simulink model "IEEE14_case"  (R2024b)
settings: Solver=FixedStepAuto  StartTime=0  StopTime=2  FixedStep=1e-7  RelTol=1e-3
values from neighbouring files (symbols this model uses):
  GFL_15_Bva = 0.009    [IEEE14_parameters.m]
  GFL_15_C_bus_pu = 7.179419    [IEEE14_parameters.m]
  GFL_15_f0 = 60    [IEEE14_parameters.m]
  GFL_15_I_id = 691.26967    [IEEE14_parameters.m]
  GFL_15_I_iq = 691.26967    [IEEE14_parameters.m]
  GFL_15_I_od = 45.2207    [IEEE14_parameters.m]
  GFL_15_I_oq = 45.2207    [IEEE14_parameters.m]
  GFL_15_I_pll = 0.78    [IEEE14_parameters.m]
  GFL_15_Kdi = 0.09    [IEEE14_parameters.m]
  GFL_15_Kdo = 0.9    [IEEE14_parameters.m]
  GFL_15_Kqi = 0.09    [IEEE14_parameters.m]
  GFL_15_Kqo = 0.9    [IEEE14_parameters.m]
  GFL_15_Lg_pu = 0.631447    [IEEE14_parameters.m]
  GFL_15_mode = 1    [IEEE14_parameters.m]
  GFL_15_P_id = 3.7166    [IEEE14_parameters.m]
  GFL_15_P_iq = 3.7166    [IEEE14_parameters.m]
  GFL_15_P_od = 0.4798    [IEEE14_parameters.m]
  GFL_15_P_oq = 0.4798    [IEEE14_parameters.m]
  GFL_15_P_pll = 290.42    [IEEE14_parameters.m]
  GFL_15_Qe_ref = 0.2    [IEEE14_parameters.m]
  GFL_15_Rg_pu = 0.024016    [IEEE14_parameters.m]
  GFL_15_Sbase = 1.000000e+4    (= 10000)    [IEEE14_parameters.m]
  GFL_15_Tdi = 0.01    [IEEE14_parameters.m]
  GFL_15_Tdo = 0.2    [IEEE14_parameters.m]
  GFL_15_Tqi = 0.01    [IEEE14_parameters.m]
  GFL_15_Tqo = 0.2    [IEEE14_parameters.m]
  GFL_15_Vbase = 380    [IEEE14_parameters.m]
  GFL_15_Vdc_ref = 1.011475    [IEEE14_parameters.m]
  GFL_15_Vdcbase = 700    [IEEE14_parameters.m]
  GFL_15_vq_ref = 0    [IEEE14_parameters.m]
  GFL_16_Bva = 0.002    [IEEE14_parameters.m]
  GFL_16_C_bus_pu = 7.179419    [IEEE14_parameters.m]
  GFL_16_f0 = 60    [IEEE14_parameters.m]
  GFL_16_I_id = 691.26967    [IEEE14_parameters.m]
  GFL_16_I_iq = 691.26967    [IEEE14_parameters.m]
  GFL_16_I_od = 45.2207    [IEEE14_parameters.m]
  GFL_16_I_oq = 45.2207    [IEEE14_parameters.m]
  GFL_16_I_pll = 0.78    [IEEE14_parameters.m]
  GFL_16_Kdi = 0.05    [IEEE14_parameters.m]
  GFL_16_Kdo = 0.5    [IEEE14_parameters.m]
  GFL_16_Kqi = 0.05    [IEEE14_parameters.m]
  GFL_16_Kqo = 0.5    [IEEE14_parameters.m]
  GFL_16_Lg_pu = 0.631447    [IEEE14_parameters.m]
  GFL_16_mode = 1    [IEEE14_parameters.m]
  GFL_16_P_id = 3.7166    [IEEE14_parameters.m]
  GFL_16_P_iq = 3.7166    [IEEE14_parameters.m]
  GFL_16_P_od = 0.4798    [IEEE14_parameters.m]
  GFL_16_P_oq = 0.4798    [IEEE14_parameters.m]
  GFL_16_P_pll = 290.42    [IEEE14_parameters.m]
  GFL_16_Qe_ref = 0.2    [IEEE14_parameters.m]
  GFL_16_Rg_pu = 0.024016    [IEEE14_parameters.m]
  GFL_16_Sbase = 1.000000e+4    (= 10000)    [IEEE14_parameters.m]
  GFL_16_Tdi = 0.01    [IEEE14_parameters.m]
  GFL_16_Tdo = 0.2    [IEEE14_parameters.m]
  GFL_16_Tqi = 0.01    [IEEE14_parameters.m]
  GFL_16_Tqo = 0.2    [IEEE14_parameters.m]
  GFL_16_Vbase = 380    [IEEE14_parameters.m]
  GFL_16_Vdc_ref = 1.01144    [IEEE14_parameters.m]
  GFL_16_Vdcbase = 700    [IEEE14_parameters.m]
  GFL_16_vq_ref = 0    [IEEE14_parameters.m]
  GFL_17_Bva = 0.002    [IEEE14_parameters.m]
  GFL_17_C_bus_pu = 7.179419    [IEEE14_parameters.m]
  GFL_17_f0 = 60    [IEEE14_parameters.m]
  GFL_17_I_id = 691.26967    [IEEE14_parameters.m]
  GFL_17_I_iq = 691.26967    [IEEE14_parameters.m]
  GFL_17_I_od = 45.2207    [IEEE14_parameters.m]
  GFL_17_I_oq = 45.2207    [IEEE14_parameters.m]
  GFL_17_I_pll = 0.78    [IEEE14_parameters.m]
  GFL_17_Kdi = 0.05    [IEEE14_parameters.m]
  GFL_17_Kdo = 0.5    [IEEE14_parameters.m]
  GFL_17_Kqi = 0.05    [IEEE14_parameters.m]
  GFL_17_Kqo = 0.5    [IEEE14_parameters.m]
  GFL_17_Lg_pu = 0.631447    [IEEE14_parameters.m]
  GFL_17_mode = 1    [IEEE14_parameters.m]
  GFL_17_P_id = 3.7166    [IEEE14_parameters.m]
  GFL_17_P_iq = 3.7166    [IEEE14_parameters.m]
  GFL_17_P_od = 0.4798    [IEEE14_parameters.m]
  GFL_17_P_oq = 0.4798    [IEEE14_parameters.m]
  GFL_17_P_pll = 290.42    [IEEE14_parameters.m]
  GFL_17_Qe_ref = 0.2    [IEEE14_parameters.m]
  GFL_17_Rg_pu = 0.024016    [IEEE14_parameters.m]
  GFL_17_Sbase = 1.000000e+4    (= 10000)    [IEEE14_parameters.m]
  GFL_17_Tdi = 0.01    [IEEE14_parameters.m]
  GFL_17_Tdo = 0.2    [IEEE14_parameters.m]
  GFL_17_Tqi = 0.01    [IEEE14_parameters.m]
  GFL_17_Tqo = 0.2    [IEEE14_parameters.m]
  GFL_17_Vbase = 380    [IEEE14_parameters.m]
  GFL_17_Vdc_ref = 1.011632    [IEEE14_parameters.m]
  GFL_17_Vdcbase = 700    [IEEE14_parameters.m]
  GFL_17_vq_ref = 0    [IEEE14_parameters.m]
  GFL_18_Bva = 0.002    [IEEE14_parameters.m]
  GFL_18_C_bus_pu = 7.179419    [IEEE14_parameters.m]
  GFL_18_f0 = 60    [IEEE14_parameters.m]
  GFL_18_I_id = 691.26967    [IEEE14_parameters.m]
  GFL_18_I_iq = 691.26967    [IEEE14_parameters.m]
  GFL_18_I_od = 45.2207    [IEEE14_parameters.m]
  GFL_18_I_oq = 45.2207    [IEEE14_parameters.m]
  GFL_18_I_pll = 0.78    [IEEE14_parameters.m]
  GFL_18_Kdi = 0.05    [IEEE14_parameters.m]
  GFL_18_Kdo = 0.5    [IEEE14_parameters.m]
  GFL_18_Kqi = 0.05    [IEEE14_parameters.m]
  GFL_18_Kqo = 0.5    [IEEE14_parameters.m]
  GFL_18_Lg_pu = 0.631447    [IEEE14_parameters.m]
  GFL_18_mode = 1    [IEEE14_parameters.m]
  GFL_18_P_id = 3.7166    [IEEE14_parameters.m]
  GFL_18_P_iq = 3.7166    [IEEE14_parameters.m]
  GFL_18_P_od = 0.4798    [IEEE14_parameters.m]
  GFL_18_P_oq = 0.4798    [IEEE14_parameters.m]
  GFL_18_P_pll = 290.42    [IEEE14_parameters.m]
  GFL_18_Qe_ref = 0.2    [IEEE14_parameters.m]
  GFL_18_Rg_pu = 0.024016    [IEEE14_parameters.m]
  GFL_18_Sbase = 1.000000e+4    (= 10000)    [IEEE14_parameters.m]
  GFL_18_Tdi = 0.01    [IEEE14_parameters.m]
  GFL_18_Tdo = 0.2    [IEEE14_parameters.m]
  GFL_18_Tqi = 0.01    [IEEE14_parameters.m]
  GFL_18_Tqo = 0.2    [IEEE14_parameters.m]
  GFL_18_Vbase = 380    [IEEE14_parameters.m]
  GFL_18_Vdc_ref = 1.011572    [IEEE14_parameters.m]
  GFL_18_Vdcbase = 700    [IEEE14_parameters.m]
  GFL_18_vq_ref = 0    [IEEE14_parameters.m]
  ... (+180 more)
(part 16 of 25)

== system IEEE14_case/SG_D_1/d_psi_d_SG_D_1_block ==
  note: d_psi_d_SG_D_1 in case14gfl
      | $2\,\pi \,f_{0}\,\left(v_{d,\mathrm{SG},D,1}\,\sin\left(\theta _{\mathrm{SG},D,1}\right)-v_{q,\mathrm{SG},D,1}\,\cos\left(\theta _{\mathrm{SG},D,1}\right)+\frac{R_{a}\,\left(\frac{\psi _{\mathrm{1d},\mathrm{SG},D,1}\,\left(x_{\mathrm{dd}}-x_{\mathrm{ddd}}\right)}{x_{\mathrm{dd}}-x_{l}}-\psi _{d,\mathrm{SG},D,1}+\frac{\psi _{\mathrm{fd},\mathrm{SG},D,1}\,\left(x_{\mathrm{ddd}}-x_{l}\right)}{x_{\mathrm{dd}}-x_{l}}\right)}{x_{\mathrm{ddd}}}+\frac{\psi _{q,\mathrm{SG},D,1}\,w_{\mathrm{SG},D,1}}{2\,f_{0}\,\pi }\right)$
      | Automatically generated on 2025-10-09 21:29:31 .
  State_psi_1d_SG_D_1_69d00 : Inport
  State_psi_d_SG_D_1_b0cbd : Inport  Port=2
  State_psi_fd_SG_D_1_aad83 : Inport  Port=3
  Input_v_d_SG_D_1_751e0 : Inport  Port=4
  State_theta_SG_D_1_5b2d6 : Inport  Port=5
  Input_v_q_SG_D_1_569c6 : Inport  Port=6
  State_theta_SG_D_1_7d7a3 : Inport  Port=7
  State_psi_q_SG_D_1_339cd : Inport  Port=8
  State_w_SG_D_1_7866a : Inport  Port=9
  Add_56184 : Sum
  Add_be544 : Sum
  Constant_-1_51278 : Constant  Value=-1
  Constant_-2.0_38dac : Constant  Value=-2.0
  Constant_2.0_c29de : Constant  Value=2.0
  Constant_R_a_cf787 : Constant  Value=R_a
  Constant_f0_76831 : Constant  Value=f0
  Constant_f0_cb811 : Constant  Value=f0
  Constant_pi_8af64 : Constant  Value=pi
  Constant_pi_fa2ea : Constant  Value=pi
  Constant_x_dd_7e7b6 : Constant  Value=x_dd
  Constant_x_dd_812da : Constant  Value=x_dd
  Constant_x_dd_b764a : Constant  Value=x_dd
  Constant_x_ddd_361c2 : Constant  Value=x_ddd
  Constant_x_ddd_731d1 : Constant  Value=x_ddd
  Constant_x_ddd_f45d6 : Constant  Value=x_ddd
  Constant_x_l_01895 : Constant  Value=x_l
  Constant_x_l_16bb1 : Constant  Value=x_l
  Constant_x_l_4d5b7 : Constant  Value=x_l
  Divide_0c8f7 : Product  Inputs=*/
  Divide_7e30b : Product  Inputs=*/
  Divide_b7777 : Product  Inputs=*/
  Divide_c3a43 : Product  Inputs=*/
  MathFunc_cos_3b064 : Trigonometry  Operator=cos
  MathFunc_sin_7ab60 : Trigonometry
  Product_22a26 : Product
  Product_40b9a : Product
  Product_4496c : Product
  Product_63206 : Product
  Product_9a24b : Product
  Product_ac20e : Product
  Product_b01b2 : Product
  Product_b1bbd : Product
  Product_b9918 : Product
  Product_d2dbc : Product
  Product_d68ab : Product
  Product_e52bf : Product
  Subtract_0ab8d : Sum  Inputs=+-
  Subtract_2360f : Sum  Inputs=+-
  Subtract_60414 : Sum  Inputs=+-
  Subtract_87491 : Sum  Inputs=+-
  Subtract_a23d2 : Sum  Inputs=+-
  Subtract_c2635 : Sum  Inputs=+-
  Subtract_ccf2d : Sum  Inputs=+-
  Blockout_d_psi_d_SG_D_1_2cdbf : Outport
  wires:
  Add_be544/1 -> Subtract_87491/1
  Product_9a24b/1 -> Divide_c3a43/1
  Subtract_ccf2d/1 -> Product_9a24b/2
  Divide_c3a43/1 -> Add_be544/1
  Product_e52bf/1 -> Product_9a24b/1
  Constant_x_ddd_361c2/1 -> Subtract_ccf2d/2
  Constant_x_dd_812da/1 -> Subtract_ccf2d/1
  State_psi_1d_SG_D_1_69d00/1 -> Product_e52bf/2
  Constant_-1_51278/1 -> Product_e52bf/1
  Product_ac20e/1 -> Divide_b7777/1
  Constant_x_l_4d5b7/1 -> Subtract_c2635/2
  State_psi_d_SG_D_1_b0cbd/1 -> Add_be544/2
  Constant_x_dd_b764a/1 -> Subtract_c2635/1
  Constant_x_ddd_731d1/1 -> Subtract_a23d2/1
  Constant_x_l_01895/1 -> Subtract_a23d2/2
  Subtract_c2635/1 -> Divide_c3a43/2
  State_psi_fd_SG_D_1_aad83/1 -> Product_ac20e/1
  Constant_x_ddd_f45d6/1 -> Divide_0c8f7/2
  Subtract_a23d2/1 -> Product_ac20e/2
  Product_d68ab/1 -> Subtract_0ab8d/2
  Constant_x_dd_7e7b6/1 -> Subtract_2360f/1
  Constant_x_l_16bb1/1 -> Subtract_2360f/2
  Subtract_2360f/1 -> Divide_b7777/2
  Divide_b7777/1 -> Subtract_87491/2
  Constant_R_a_cf787/1 -> Product_63206/1
  Subtract_87491/1 -> Product_63206/2
  MathFunc_cos_3b064/1 -> Product_4496c/2
  State_theta_SG_D_1_5b2d6/1 -> MathFunc_sin_7ab60/1
  Divide_0c8f7/1 -> Subtract_0ab8d/1
  Product_63206/1 -> Divide_0c8f7/1
  MathFunc_sin_7ab60/1 -> Product_d68ab/2
  Input_v_d_SG_D_1_751e0/1 -> Product_d68ab/1
  Product_b9918/1 -> Blockout_d_psi_d_SG_D_1_2cdbf/1
  Product_d2dbc/1 -> Product_b9918/1
  Product_22a26/1 -> Product_d2dbc/1
  State_theta_SG_D_1_7d7a3/1 -> MathFunc_cos_3b064/1
  Constant_2.0_c29de/1 -> Product_40b9a/1
  Constant_pi_fa2ea/1 -> Product_40b9a/2
  Input_v_q_SG_D_1_569c6/1 -> Product_4496c/1
  Constant_f0_76831/1 -> Product_d2dbc/2
  State_psi_q_SG_D_1_339cd/1 -> Product_b1bbd/1
  State_w_SG_D_1_7866a/1 -> Product_b1bbd/2
  Product_40b9a/1 -> Product_b01b2/1
  Constant_pi_8af64/1 -> Product_22a26/2
  Constant_f0_cb811/1 -> Product_b01b2/2
  Constant_-2.0_38dac/1 -> Product_22a26/1
  Add_56184/1 -> Subtract_60414/1
  Subtract_0ab8d/1 -> Add_56184/1
  Product_4496c/1 -> Add_56184/2
  Product_b1bbd/1 -> Divide_7e30b/1
  Product_b01b2/1 -> Divide_7e30b/2
  Divide_7e30b/1 -> Subtract_60414/2
  Subtract_60414/1 -> Product_b9918/2

== system IEEE14_case/SG_D_1/d_psi_fd_SG_D_1_block ==
  note: d_psi_fd_SG_D_1 in case14gfl
      | $-\frac{\psi _{\mathrm{fd},\mathrm{SG},D,1}-E_{\mathrm{fd},\mathrm{SG},D,1}+\left(x_{d}-x_{\mathrm{dd}}\right)\,\left(\frac{\frac{\psi _{\mathrm{1d},\mathrm{SG},D,1}\,\left(x_{\mathrm{dd}}-x_{\mathrm{ddd}}\right)}{x_{\mathrm{dd}}-x_{l}}-\psi _{d,\mathrm{SG},D,1}+\frac{\psi _{\mathrm{fd},\mathrm{SG},D,1}\,\left(x_{\mathrm{ddd}}-x_{l}\right)}{x_{\mathrm{dd}}-x_{l}}}{x_{\mathrm{ddd}}}-\frac{\left(x_{\mathrm{dd}}-x_{\mathrm{ddd}}\right)\,\left(\psi _{\mathrm{1d},\mathrm{SG},D,1}-\psi _{\mathrm{fd},\mathrm{SG},D,1}+\frac{\left(x_{\mathrm{dd}}-x_{l}\right)\,\left(\frac{\psi _{\mathrm{1d},\mathrm{SG},D,1}\,\left(x_{\mathrm{dd}}-x_{\mathrm{ddd}}\right)}{x_{\mathrm{dd}}-x_{l}}-\psi _{d,\mathrm{SG},D,1}+\frac{\psi _{\mathrm{fd},\mathrm{SG},D,1}\,\left(x_{\mathrm{ddd}}-x_{l}\right)}{x_{\mathrm{dd}}-x_{l}}\right)}{x_{\mathrm{ddd}}}\right)}{{\left(x_{\mathrm{dd}}-x_{l}\right)}^2}\right)}{T_{\mathrm{dd}}}$
      | Automatically generated on 2025-10-09 21:29:56 .
  State_E_fd_SG_D_1_05819 : Inport
  State_psi_fd_SG_D_1_8f7d3 : Inport  Port=2
  State_psi_1d_SG_D_1_1898e : Inport  Port=3
  State_psi_fd_SG_D_1_d976b : Inport  Port=4
  State_psi_1d_SG_D_1_f6ad7 : Inport  Port=5
  State_psi_d_SG_D_1_eef22 : Inport  Port=6
  State_psi_fd_SG_D_1_c7a2f : Inport  Port=7
  State_psi_1d_SG_D_1_2c9f9 : Inport  Port=8
  State_psi_d_SG_D_1_5418d : Inport  Port=9
  State_psi_fd_SG_D_1_86724 : Inport  Port=10
  Add_0e10e : Sum
  Add_855f0 : Sum
  Constant_-1_2c57e : Constant  Value=-1
  Constant_-1_a28a2 : Constant  Value=-1
  Constant_-1_c60db : Constant  Value=-1
  Constant_2.0_ead1b : Constant  Value=2.0
  Constant_T_dd_4fac4 : Constant  Value=T_dd
  Constant_x_d_dd175 : Constant  Value=x_d
  Constant_x_dd_048c0 : Constant  Value=x_dd
  Constant_x_dd_0c681 : Constant  Value=x_dd
  Constant_x_dd_17d74 : Constant  Value=x_dd
  Constant_x_dd_1bbdd : Constant  Value=x_dd
  Constant_x_dd_2d3b2 : Constant  Value=x_dd
  Constant_x_dd_32bd9 : Constant  Value=x_dd
  Constant_x_dd_778d2 : Constant  Value=x_dd
  Constant_x_dd_c0a9a : Constant  Value=x_dd
  Constant_x_dd_d296d : Constant  Value=x_dd
  Constant_x_dd_f5264 : Constant  Value=x_dd
  Constant_x_ddd_147e2 : Constant  Value=x_ddd
  Constant_x_ddd_27727 : Constant  Value=x_ddd
  Constant_x_ddd_30073 : Constant  Value=x_ddd
  Constant_x_ddd_77236 : Constant  Value=x_ddd
  Constant_x_ddd_7c972 : Constant  Value=x_ddd
  Constant_x_ddd_8e231 : Constant  Value=x_ddd
  Constant_x_ddd_dc7b0 : Constant  Value=x_ddd
  Constant_x_l_2ab6b : Constant  Value=x_l
  Constant_x_l_30b80 : Constant  Value=x_l
  Constant_x_l_71782 : Constant  Value=x_l
  Constant_x_l_74cf2 : Constant  Value=x_l
  Constant_x_l_98a55 : Constant  Value=x_l
  Constant_x_l_9e494 : Constant  Value=x_l
  Constant_x_l_a6392 : Constant  Value=x_l
  Constant_x_l_beb3a : Constant  Value=x_l
  Divide_01689 : Product  Inputs=*/
  Divide_0f83a : Product  Inputs=*/
  Divide_6a9fb : Product  Inputs=*/
  Divide_7fd4b : Product  Inputs=*/
  Divide_9001b : Product  Inputs=*/
  Divide_a851a : Product  Inputs=*/
  Divide_b92f6 : Product  Inputs=*/
  Divide_fdf02 : Product  Inputs=*/
  Power_7840a : Math  Operator=pow
  Product_16821 : Product
  Product_1a66a : Product
  Product_2f431 : Product
  Product_6b392 : Product
  Product_7d54a : Product
  Product_b5b20 : Product
  Product_b5cc8 : Product
  Product_b7127 : Product
  Product_d3415 : Product
  Product_f7a96 : Product
  Subtract_0cd1e : Sum  Inputs=+-
  Subtract_2a961 : Sum  Inputs=+-
  Subtract_3bb19 : Sum  Inputs=+-
  Subtract_4453c : Sum  Inputs=+-
  Subtract_469f7 : Sum  Inputs=+-
  Subtract_562ce : Sum  Inputs=+-
  Subtract_63680 : Sum  Inputs=+-
  Subtract_65ab3 : Sum  Inputs=+-
  Subtract_6a7c7 : Sum  Inputs=+-
  Subtract_6faa6 : Sum  Inputs=+-
  Subtract_72a4d : Sum  Inputs=+-
  Subtract_73178 : Sum  Inputs=+-
  Subtract_80272 : Sum  Inputs=+-
  Subtract_9f379 : Sum  Inputs=+-
  Subtract_b24c4 : Sum  Inputs=+-
  Subtract_b29f2 : Sum  Inputs=+-
  Subtract_cbbe3 : Sum  Inputs=+-
  Subtract_db76e : Sum  Inputs=+-
  Subtract_ff79e : Sum  Inputs=+-
  Blockout_d_psi_fd_SG_D_1_936e9 : Outport
  wires:
  State_psi_d_SG_D_1_eef22/1 -> Add_855f0/2
  Constant_x_dd_17d74/1 -> Subtract_73178/1
  Product_2f431/1 -> Divide_01689/1
  Subtract_65ab3/1 -> Product_2f431/2
  Subtract_6faa6/1 -> Product_d3415/2
  Product_b5b20/1 -> Product_2f431/1
  Constant_x_dd_f5264/1 -> Subtract_65ab3/1
  Constant_x_l_30b80/1 -> Subtract_3bb19/2
  Constant_-1_2c57e/1 -> Product_b5b20/1
  Subtract_3bb19/1 -> Product_d3415/1
  Constant_x_l_71782/1 -> Subtract_73178/2
  Constant_x_ddd_27727/1 -> Subtract_65ab3/2
  State_psi_1d_SG_D_1_f6ad7/1 -> Product_b5b20/2
  Constant_x_ddd_dc7b0/1 -> Subtract_63680/1
  Constant_x_l_a6392/1 -> Subtract_63680/2
  State_E_fd_SG_D_1_05819/1 -> Subtract_2a961/1
  Divide_01689/1 -> Add_855f0/1
  Subtract_73178/1 -> Divide_01689/2
  State_psi_fd_SG_D_1_c7a2f/1 -> Product_1a66a/1
  Constant_x_ddd_8e231/1 -> Divide_7fd4b/2
  Subtract_63680/1 -> Product_1a66a/2
  Constant_x_dd_1bbdd/1 -> Subtract_4453c/1
  Constant_x_dd_048c0/1 -> Subtract_0cd1e/1
  State_psi_fd_SG_D_1_8f7d3/1 -> Subtract_2a961/2
  Constant_x_l_2ab6b/1 -> Subtract_4453c/2
  Product_1a66a/1 -> Divide_b92f6/1
  Constant_-1_c60db/1 -> Product_b5cc8/1
  Subtract_4453c/1 -> Divide_b92f6/2
  Constant_x_dd_d296d/1 -> Subtract_3bb19/1
  Add_855f0/1 -> Subtract_6faa6/1
  Constant_x_l_9e494/1 -> Subtract_0cd1e/2
  Divide_b92f6/1 -> Subtract_6faa6/2
  Divide_0f83a/1 -> Subtract_9f379/1
  Constant_-1_a28a2/1 -> Product_7d54a/1
  State_psi_1d_SG_D_1_2c9f9/1 -> Product_7d54a/2
  Constant_x_dd_c0a9a/1 -> Subtract_db76e/1
  Subtract_80272/1 -> Product_b5cc8/2
  Constant_x_ddd_30073/1 -> Subtract_db76e/2
  Product_7d54a/1 -> Product_16821/1
  Constant_2.0_ead1b/1 -> Power_7840a/2
  Product_16821/1 -> Divide_9001b/1
  Subtract_9f379/1 -> Product_6b392/2
  Subtract_db76e/1 -> Product_16821/2
  State_psi_d_SG_D_1_5418d/1 -> Add_0e10e/2
  Constant_x_dd_32bd9/1 -> Subtract_6a7c7/1
  Constant_x_l_beb3a/1 -> Subtract_6a7c7/2
  Constant_x_dd_0c681/1 -> Subtract_80272/1
  Divide_7fd4b/1 -> Subtract_562ce/2
  Constant_x_ddd_147e2/1 -> Subtract_b29f2/1
  Constant_x_ddd_7c972/1 -> Subtract_80272/2
  Constant_x_l_98a55/1 -> Subtract_b29f2/2
  Subtract_b29f2/1 -> Product_f7a96/2
  State_psi_1d_SG_D_1_1898e/1 -> Subtract_cbbe3/1
  Product_f7a96/1 -> Divide_6a9fb/1
  State_psi_fd_SG_D_1_d976b/1 -> Subtract_cbbe3/2
  State_psi_fd_SG_D_1_86724/1 -> Product_f7a96/1
  Product_d3415/1 -> Divide_7fd4b/1
  Divide_9001b/1 -> Add_0e10e/1
  Subtract_6a7c7/1 -> Divide_9001b/2
  Constant_x_dd_778d2/1 -> Subtract_72a4d/1
  Constant_x_l_74cf2/1 -> Subtract_72a4d/2
  Divide_6a9fb/1 -> Subtract_ff79e/2
  Subtract_cbbe3/1 -> Subtract_562ce/1
  Subtract_72a4d/1 -> Divide_6a9fb/2
  Subtract_562ce/1 -> Product_b7127/2
  Product_b5cc8/1 -> Product_b7127/1
  Subtract_0cd1e/1 -> Power_7840a/1
  Add_0e10e/1 -> Subtract_ff79e/1
  Product_b7127/1 -> Divide_0f83a/1
  Power_7840a/1 -> Divide_0f83a/2
  Subtract_ff79e/1 -> Divide_a851a/1
  Constant_x_ddd_77236/1 -> Divide_a851a/2
  Constant_x_d_dd175/1 -> Subtract_469f7/1
  Constant_x_dd_2d3b2/1 -> Subtract_469f7/2
  Divide_a851a/1 -> Subtract_9f379/2
  Subtract_469f7/1 -> Product_6b392/1
  Subtract_2a961/1 -> Subtract_b24c4/1
  Product_6b392/1 -> Subtract_b24c4/2
  Subtract_b24c4/1 -> Divide_fdf02/1
  Constant_T_dd_4fac4/1 -> Divide_fdf02/2
  Divide_fdf02/1 -> Blockout_d_psi_fd_SG_D_1_936e9/1

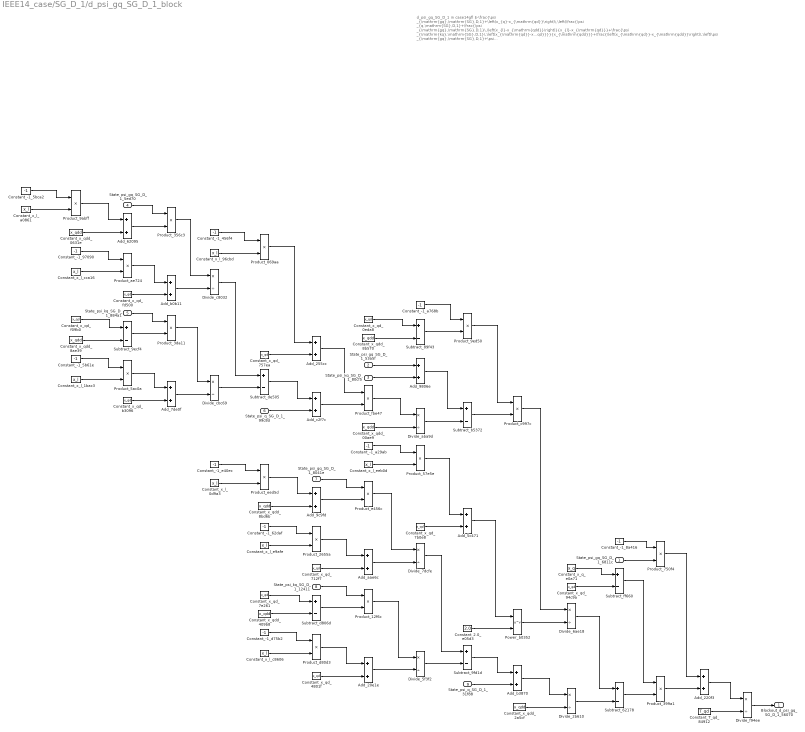
== system IEEE14_case/SG_D_1/d_psi_gq_SG_D_1_block ==
  note: d_psi_gq_SG_D_1 in case14gfl
      | $-\frac{\psi _{\mathrm{gq},\mathrm{SG},D,1}+\left(x_{q}-x_{\mathrm{qd}}\right)\,\left(\frac{\psi _{q,\mathrm{SG},D,1}+\frac{\psi _{\mathrm{gq},\mathrm{SG},D,1}\,\left(x_{l}-x_{\mathrm{qdd}}\right)}{x_{l}-x_{\mathrm{qd}}}+\frac{\psi _{\mathrm{kq},\mathrm{SG},D,1}\,\left(x_{\mathrm{qd}}-x_{\mathrm{qdd}}\right)}{x_{l}-x_{\mathrm{qd}}}}{x_{\mathrm{qdd}}}+\frac{\left(x_{\mathrm{qd}}-x_{\mathrm{qdd}}\right)\,\left(\psi _{\mathrm{gq},\mathrm{SG},D,1}+\psi _{\mathrm{kq},\mathrm{SG},D,1}+\frac{\left(x_{l}-x_{\mathrm{qd}}\right)\,\left(\psi _{q,\mathrm{SG},D,1}+\frac{\psi _{\mathrm{gq},\mathrm{SG},D,1}\,\left(x_{l}-x_{\mathrm{qdd}}\right)}{x_{l}-x_{\mathrm{qd}}}+\frac{\psi _{\mathrm{kq},\mathrm{SG},D,1}\,\left(x_{\mathrm{qd}}-x_{\mathrm{qdd}}\right)}{x_{l}-x_{\mathrm{qd}}}\right)}{x_{\mathrm{qdd}}}\right)}{{\left(x_{l}-x_{\mathrm{qd}}\right)}^2}\right)}{T_{\mathrm{qd}}}$
      | Automatically generated on 2025-10-09 21:30:03 .
  State_psi_gq_SG_D_1_6811c : Inport
  State_psi_gq_SG_D_1_53a5f : Inport  Port=2
  State_psi_kq_SG_D_1_80cf5 : Inport  Port=3
  State_psi_gq_SG_D_1_5ed70 : Inport  Port=4
  State_psi_kq_SG_D_1_884a1 : Inport  Port=5
  State_psi_q_SG_D_1_99c8d : Inport  Port=6
  State_psi_gq_SG_D_1_8041e : Inport  Port=7
  State_psi_kq_SG_D_1_12411 : Inport  Port=8
  State_psi_q_SG_D_1_31f88 : Inport  Port=9
  Add_20e1e : Sum
  Add_220f3 : Sum
  Add_255cc : Sum
  Add_5c471 : Sum
  Add_62095 : Sum
  Add_7de0f : Sum
  Add_9806e : Sum
  Add_9c9fd : Sum
  Add_aae6c : Sum
  Add_b0b11 : Sum
  Add_b3870 : Sum
  Add_c2f7c : Sum
  Constant_-1_456f4 : Constant  Value=-1
  Constant_-1_5b61e : Constant  Value=-1
  Constant_-1_5bca2 : Constant  Value=-1
  Constant_-1_62daf : Constant  Value=-1
  Constant_-1_8a416 : Constant  Value=-1
  Constant_-1_97090 : Constant  Value=-1
  Constant_-1_a29ab : Constant  Value=-1
  Constant_-1_a768b : Constant  Value=-1
  Constant_-1_d75b2 : Constant  Value=-1
  Constant_-1_e40ec : Constant  Value=-1
  Constant_2.0_e05d3 : Constant  Value=2.0
  Constant_T_qd_84912 : Constant  Value=T_qd
  Constant_x_l_0d9a3 : Constant  Value=x_l
  Constant_x_l_1bac3 : Constant  Value=x_l
  Constant_x_l_96cbd : Constant  Value=x_l
  Constant_x_l_a0861 : Constant  Value=x_l
  Constant_x_l_c8606 : Constant  Value=x_l
  Constant_x_l_cca16 : Constant  Value=x_l
  Constant_x_l_e9afe : Constant  Value=x_l
  Constant_x_l_eeb0d : Constant  Value=x_l
  Constant_x_q_e0a71 : Constant  Value=x_q
  Constant_x_qd_0eda8 : Constant  Value=x_qd
  Constant_x_qd_4801f : Constant  Value=x_qd
  Constant_x_qd_712f7 : Constant  Value=x_qd
  Constant_x_qd_757ea : Constant  Value=x_qd
  Constant_x_qd_7b0e8 : Constant  Value=x_qd
  Constant_x_qd_7e261 : Constant  Value=x_qd
  Constant_x_qd_94c9a : Constant  Value=x_qd
  Constant_x_qd_b3096 : Constant  Value=x_qd
  Constant_x_qd_f09b0 : Constant  Value=x_qd
  Constant_x_qd_fd500 : Constant  Value=x_qd
  Constant_x_qdd_00ae9 : Constant  Value=x_qdd
  Constant_x_qdd_0631e : Constant  Value=x_qdd
  Constant_x_qdd_2a5cf : Constant  Value=x_qdd
  Constant_x_qdd_409b8 : Constant  Value=x_qdd
  Constant_x_qdd_8ae39 : Constant  Value=x_qdd
  Constant_x_qdd_8b570 : Constant  Value=x_qdd
  Constant_x_qdd_8bd6b : Constant  Value=x_qdd
  Divide_2b610 : Product  Inputs=*/
  Divide_5f3f2 : Product  Inputs=*/
  Divide_6ae18 : Product  Inputs=*/
  Divide_7dcfe : Product  Inputs=*/
  Divide_aba9d : Product  Inputs=*/
  Divide_c8032 : Product  Inputs=*/
  Divide_cbc69 : Product  Inputs=*/
  Divide_f94ee : Product  Inputs=*/
  Power_b0352 : Math  Operator=pow
  Product_069aa : Product
  Product_12f6c : Product
  Product_2655a : Product
  Product_356c3 : Product
  Product_399a1 : Product
  Product_3da11 : Product
  Product_57e5e : Product
  Product_5ac0a : Product
  Product_750f4 : Product
  Product_9abff : Product
  Product_9ed50 : Product
  Product_ae724 : Product
  Product_c997c : Product
  Product_d80d3 : Product
  Product_e456c : Product
  Product_eed5d : Product
  Product_fbe47 : Product
  Subtract_62178 : Sum  Inputs=+-
  Subtract_89f43 : Sum  Inputs=+-
  Subtract_9ecf4 : Sum  Inputs=+-
  Subtract_9fd1d : Sum  Inputs=+-
  Subtract_b5372 : Sum  Inputs=+-
  Subtract_d806d : Sum  Inputs=+-
  Subtract_de505 : Sum  Inputs=+-
  Subtract_ff660 : Sum  Inputs=+-
  Blockout_d_psi_gq_SG_D_1_56070 : Outport
  wires:
  State_psi_gq_SG_D_1_5ed70/1 -> Product_356c3/1
  Constant_-1_97090/1 -> Product_ae724/1
  Divide_c8032/1 -> Subtract_de505/1
  Add_b0b11/1 -> Divide_c8032/2
  Product_9abff/1 -> Add_62095/1
  Constant_x_qd_757ea/1 -> Add_255cc/2
  Constant_-1_5bca2/1 -> Product_9abff/1
  Constant_x_qdd_0631e/1 -> Add_62095/2
  Constant_x_l_cca16/1 -> Product_ae724/2
  Constant_x_l_a0861/1 -> Product_9abff/2
  Constant_-1_5b61e/1 -> Product_5ac0a/1
  Constant_x_qd_f09b0/1 -> Subtract_9ecf4/1
  Constant_x_qdd_00ae9/1 -> Divide_aba9d/2
  Constant_x_l_1bac3/1 -> Product_5ac0a/2
  Constant_x_qdd_8ae39/1 -> Subtract_9ecf4/2
  Subtract_de505/1 -> Add_c2f7c/1
  Add_62095/1 -> Product_356c3/2
  Product_356c3/1 -> Divide_c8032/1
  Product_ae724/1 -> Add_b0b11/1
  Constant_x_qd_fd500/1 -> Add_b0b11/2
  State_psi_kq_SG_D_1_884a1/1 -> Product_3da11/1
  Product_5ac0a/1 -> Add_7de0f/1
  Subtract_9ecf4/1 -> Product_3da11/2
  Constant_x_qd_b3096/1 -> Add_7de0f/2
  Product_3da11/1 -> Divide_cbc69/1
  Add_7de0f/1 -> Divide_cbc69/2
  Constant_-1_a768b/1 -> Product_9ed50/1
  Constant_-1_456f4/1 -> Product_069aa/1
  Add_aae6c/1 -> Divide_7dcfe/2
  Product_d80d3/1 -> Add_20e1e/1
  Subtract_d806d/1 -> Product_12f6c/2
  Constant_x_l_96cbd/1 -> Product_069aa/2
  Divide_cbc69/1 -> Subtract_de505/2
  Subtract_ff660/1 -> Product_399a1/1
  Constant_-1_a29ab/1 -> Product_57e5e/1
  Constant_-1_e40ec/1 -> Product_eed5d/1
  Constant_x_l_eeb0d/1 -> Product_57e5e/2
  Constant_x_l_0d9a3/1 -> Product_eed5d/2
  Constant_x_qd_712f7/1 -> Add_aae6c/2
  Product_069aa/1 -> Add_255cc/1
  State_psi_q_SG_D_1_99c8d/1 -> Add_c2f7c/2
  Product_eed5d/1 -> Add_9c9fd/1
  Constant_x_qdd_8bd6b/1 -> Add_9c9fd/2
  Constant_-1_62daf/1 -> Product_2655a/1
  Constant_x_qd_4801f/1 -> Add_20e1e/2
  Add_255cc/1 -> Product_fbe47/1
  Constant_x_l_e9afe/1 -> Product_2655a/2
  Constant_-1_d75b2/1 -> Product_d80d3/1
  Constant_x_qd_7e261/1 -> Subtract_d806d/1
  Product_fbe47/1 -> Divide_aba9d/1
  Constant_x_l_c8606/1 -> Product_d80d3/2
  Divide_6ae18/1 -> Subtract_62178/1
  Constant_x_qdd_409b8/1 -> Subtract_d806d/2
  Add_c2f7c/1 -> Product_fbe47/2
  State_psi_gq_SG_D_1_8041e/1 -> Product_e456c/1
  Add_9c9fd/1 -> Product_e456c/2
  Product_2655a/1 -> Add_aae6c/1
  State_psi_kq_SG_D_1_12411/1 -> Product_12f6c/1
  Add_20e1e/1 -> Divide_5f3f2/2
  State_psi_gq_SG_D_1_53a5f/1 -> Add_9806e/1
  Constant_x_qd_0eda8/1 -> Subtract_89f43/1
  Constant_x_qdd_8b570/1 -> Subtract_89f43/2
  Product_12f6c/1 -> Divide_5f3f2/1
  State_psi_kq_SG_D_1_80cf5/1 -> Add_9806e/2
  Product_e456c/1 -> Divide_7dcfe/1
  Subtract_89f43/1 -> Product_9ed50/2
  Add_9806e/1 -> Subtract_b5372/1
  Divide_aba9d/1 -> Subtract_b5372/2
  Product_57e5e/1 -> Add_5c471/1
  Constant_x_qd_7b0e8/1 -> Add_5c471/2
  Divide_7dcfe/1 -> Subtract_9fd1d/1
  Divide_5f3f2/1 -> Subtract_9fd1d/2
  Product_9ed50/1 -> Product_c997c/1
  Subtract_b5372/1 -> Product_c997c/2
  Add_5c471/1 -> Power_b0352/1
  Constant_2.0_e05d3/1 -> Power_b0352/2
  Subtract_9fd1d/1 -> Add_b3870/1
  State_psi_q_SG_D_1_31f88/1 -> Add_b3870/2
  Product_c997c/1 -> Divide_6ae18/1
  Power_b0352/1 -> Divide_6ae18/2
  Add_b3870/1 -> Divide_2b610/1
  Constant_x_qdd_2a5cf/1 -> Divide_2b610/2
  Constant_x_q_e0a71/1 -> Subtract_ff660/1
  Constant_x_qd_94c9a/1 -> Subtract_ff660/2
  Divide_2b610/1 -> Subtract_62178/2
  Constant_-1_8a416/1 -> Product_750f4/1
  State_psi_gq_SG_D_1_6811c/1 -> Product_750f4/2
  Subtract_62178/1 -> Product_399a1/2
  Product_750f4/1 -> Add_220f3/1
  Product_399a1/1 -> Add_220f3/2
  Add_220f3/1 -> Divide_f94ee/1
  Constant_T_qd_84912/1 -> Divide_f94ee/2
  Divide_f94ee/1 -> Blockout_d_psi_gq_SG_D_1_56070/1

== system IEEE14_case/SG_D_1/d_psi_kq_SG_D_1_block ==
  note: d_psi_kq_SG_D_1 in case14gfl
      | $-\frac{\psi _{\mathrm{gq},\mathrm{SG},D,1}+\psi _{\mathrm{kq},\mathrm{SG},D,1}+\frac{\left(x_{l}-x_{\mathrm{qd}}\right)\,\left(\psi _{q,\mathrm{SG},D,1}+\frac{\psi _{\mathrm{gq},\mathrm{SG},D,1}\,\left(x_{l}-x_{\mathrm{qdd}}\right)}{x_{l}-x_{\mathrm{qd}}}+\frac{\psi _{\mathrm{kq},\mathrm{SG},D,1}\,\left(x_{\mathrm{qd}}-x_{\mathrm{qdd}}\right)}{x_{l}-x_{\mathrm{qd}}}\right)}{x_{\mathrm{qdd}}}}{T_{\mathrm{qdd}}}$
      | Automatically generated on 2025-10-09 21:30:06 .
  State_psi_gq_SG_D_1_dba3b : Inport
  State_psi_kq_SG_D_1_b5070 : Inport  Port=2
  State_psi_gq_SG_D_1_cd69f : Inport  Port=3
  State_psi_kq_SG_D_1_7d6ac : Inport  Port=4
  State_psi_q_SG_D_1_c6187 : Inport  Port=5
  Add_21b09 : Sum
  Add_68b64 : Sum
  Add_9c914 : Sum
  Add_b2281 : Sum
  Add_b7d09 : Sum
  Add_e973c : Sum
  Constant_-1_00bfa : Constant  Value=-1
  Constant_-1_179e3 : Constant  Value=-1
  Constant_-1_85ee2 : Constant  Value=-1
  Constant_-1_ceb72 : Constant  Value=-1
  Constant_-1_f75a4 : Constant  Value=-1
  Constant_T_qdd_671ca : Constant  Value=T_qdd
  Constant_x_l_09b47 : Constant  Value=x_l
  Constant_x_l_3dd12 : Constant  Value=x_l
  Constant_x_l_594db : Constant  Value=x_l
  Constant_x_l_90045 : Constant  Value=x_l
  Constant_x_qd_28365 : Constant  Value=x_qd
  Constant_x_qd_39bbe : Constant  Value=x_qd
  Constant_x_qd_4d59d : Constant  Value=x_qd
  Constant_x_qd_e67c6 : Constant  Value=x_qd
  Constant_x_qdd_441e4 : Constant  Value=x_qdd
  Constant_x_qdd_5f5fc : Constant  Value=x_qdd
  Constant_x_qdd_f248a : Constant  Value=x_qdd
  Divide_a0dae : Product  Inputs=*/
  Divide_cf612 : Product  Inputs=*/
  Divide_dc61d : Product  Inputs=*/
  Divide_e2f45 : Product  Inputs=*/
  Product_5c33e : Product
  Product_9c1da : Product
  Product_b3437 : Product
  Product_cd955 : Product
  Product_cdcc9 : Product
  Product_d5255 : Product
  Product_e33de : Product
  Product_e9ac0 : Product
  Subtract_1b184 : Sum  Inputs=+-
  Subtract_884b7 : Sum  Inputs=+-
  Subtract_bce37 : Sum  Inputs=+-
  Blockout_d_psi_kq_SG_D_1_d51b4 : Outport
  wires:
  Product_9c1da/1 -> Add_e973c/1
  Constant_-1_ceb72/1 -> Product_9c1da/1
  Constant_x_l_09b47/1 -> Product_9c1da/2
  Constant_x_qdd_441e4/1 -> Add_e973c/2
  Constant_-1_179e3/1 -> Product_cd955/1
  Constant_x_qd_e67c6/1 -> Subtract_bce37/1
  Constant_x_qd_28365/1 -> Add_b7d09/2
  Constant_-1_00bfa/1 -> Product_b3437/1
  Constant_x_l_3dd12/1 -> Product_cd955/2
  Constant_x_qdd_f248a/1 -> Subtract_bce37/2
  Constant_x_qd_39bbe/1 -> Add_68b64/2
  Constant_x_l_594db/1 -> Product_b3437/2
  Subtract_1b184/1 -> Add_21b09/1
  Product_e33de/1 -> Subtract_1b184/1
  State_psi_gq_SG_D_1_cd69f/1 -> Product_5c33e/1
  Add_e973c/1 -> Product_5c33e/2
  Product_b3437/1 -> Add_b2281/1
  Constant_x_qd_4d59d/1 -> Add_b2281/2
  State_psi_kq_SG_D_1_7d6ac/1 -> Product_d5255/1
  Product_cd955/1 -> Add_68b64/1
  Subtract_bce37/1 -> Product_d5255/2
  Product_5c33e/1 -> Divide_e2f45/1
  Add_b2281/1 -> Divide_e2f45/2
  Product_d5255/1 -> Divide_cf612/1
  Add_68b64/1 -> Divide_cf612/2
  Constant_-1_f75a4/1 -> Product_e9ac0/1
  Constant_x_l_90045/1 -> Product_e9ac0/2
  Divide_e2f45/1 -> Subtract_884b7/1
  Divide_cf612/1 -> Subtract_884b7/2
  Product_e9ac0/1 -> Add_b7d09/1
  Add_9c914/1 -> Product_cdcc9/2
  Subtract_884b7/1 -> Add_9c914/1
  State_psi_q_SG_D_1_c6187/1 -> Add_9c914/2
  Constant_-1_85ee2/1 -> Product_e33de/1
  State_psi_gq_SG_D_1_dba3b/1 -> Product_e33de/2
  Divide_dc61d/1 -> Add_21b09/2
  Product_cdcc9/1 -> Divide_dc61d/1
  Add_b7d09/1 -> Product_cdcc9/1
  State_psi_kq_SG_D_1_b5070/1 -> Subtract_1b184/2
  Constant_x_qdd_5f5fc/1 -> Divide_dc61d/2
  Add_21b09/1 -> Divide_a0dae/1
  Constant_T_qdd_671ca/1 -> Divide_a0dae/2
  Divide_a0dae/1 -> Blockout_d_psi_kq_SG_D_1_d51b4/1

== system IEEE14_case/SG_D_1/d_psi_q_SG_D_1_block ==
  note: d_psi_q_SG_D_1 in case14gfl
      | $2\,\pi \,f_{0}\,\left(v_{d,\mathrm{SG},D,1}\,\cos\left(\theta _{\mathrm{SG},D,1}\right)+v_{q,\mathrm{SG},D,1}\,\sin\left(\theta _{\mathrm{SG},D,1}\right)-\frac{R_{a}\,\left(\psi _{q,\mathrm{SG},D,1}+\frac{\psi _{\mathrm{gq},\mathrm{SG},D,1}\,\left(x_{l}-x_{\mathrm{qdd}}\right)}{x_{l}-x_{\mathrm{qd}}}+\frac{\psi _{\mathrm{kq},\mathrm{SG},D,1}\,\left(x_{\mathrm{qd}}-x_{\mathrm{qdd}}\right)}{x_{l}-x_{\mathrm{qd}}}\right)}{x_{\mathrm{qdd}}}-\frac{\psi _{d,\mathrm{SG},D,1}\,w_{\mathrm{SG},D,1}}{2\,f_{0}\,\pi }\right)$
      | Automatically generated on 2025-10-09 21:29:51 .
  State_psi_gq_SG_D_1_af930 : Inport
  State_psi_kq_SG_D_1_494df : Inport  Port=2
  State_psi_q_SG_D_1_68044 : Inport  Port=3
  Input_v_d_SG_D_1_3462f : Inport  Port=4
  State_theta_SG_D_1_16401 : Inport  Port=5
  Input_v_q_SG_D_1_86d27 : Inport  Port=6
  State_theta_SG_D_1_4261b : Inport  Port=7
  State_psi_d_SG_D_1_ad817 : Inport  Port=8
  State_w_SG_D_1_856b5 : Inport  Port=9
  Add_16bac : Sum
  Add_3c619 : Sum
  Add_3fe38 : Sum
  Add_7d812 : Sum
  Add_97b80 : Sum
  Constant_-1_7053a : Constant  Value=-1
  Constant_-1_922f9 : Constant  Value=-1
  Constant_-1_b6810 : Constant  Value=-1
  Constant_-2.0_8fd1c : Constant  Value=-2.0
  Constant_2.0_360c5 : Constant  Value=2.0
  Constant_R_a_cb351 : Constant  Value=R_a
  Constant_f0_165d7 : Constant  Value=f0
  Constant_f0_dc23e : Constant  Value=f0
  Constant_pi_8069f : Constant  Value=pi
  Constant_pi_80d9b : Constant  Value=pi
  Constant_x_l_6e0a2 : Constant  Value=x_l
  Constant_x_l_b28d6 : Constant  Value=x_l
  Constant_x_l_c3d6c : Constant  Value=x_l
  Constant_x_qd_2eb8b : Constant  Value=x_qd
  Constant_x_qd_82ebf : Constant  Value=x_qd
  Constant_x_qd_f92bb : Constant  Value=x_qd
  Constant_x_qdd_69022 : Constant  Value=x_qdd
  Constant_x_qdd_d1603 : Constant  Value=x_qdd
  Constant_x_qdd_d808c : Constant  Value=x_qdd
  Divide_0cb61 : Product  Inputs=*/
  Divide_2b1a9 : Product  Inputs=*/
  Divide_4c773 : Product  Inputs=*/
  Divide_fa36b : Product  Inputs=*/
  MathFunc_cos_1cdd6 : Trigonometry  Operator=cos
  MathFunc_sin_c5f98 : Trigonometry
  Product_1b672 : Product
  Product_1c24e : Product
  Product_26d1a : Product
  Product_2f737 : Product
  Product_39025 : Product
  Product_578ea : Product
  Product_5e589 : Product
  Product_a14b6 : Product
  Product_bc97e : Product
  Product_c62d3 : Product
  Product_cb3f5 : Product
  Product_dbf66 : Product
  Product_f7217 : Product
  Product_fa442 : Product
  Subtract_3f2ba : Sum  Inputs=+-
  Subtract_754fd : Sum  Inputs=+-
  Subtract_ba1bd : Sum  Inputs=+-
  Subtract_d1edb : Sum  Inputs=+-
  Blockout_d_psi_q_SG_D_1_f8953 : Outport
  wires:
  Divide_2b1a9/1 -> Subtract_ba1bd/1
  Product_2f737/1 -> Add_97b80/1
  Constant_x_l_b28d6/1 -> Product_2f737/2
  Constant_-1_7053a/1 -> Product_2f737/1
  Constant_x_qdd_d808c/1 -> Add_97b80/2
  Constant_x_l_6e0a2/1 -> Product_1c24e/2
  Constant_-1_922f9/1 -> Product_1c24e/1
  Constant_x_l_c3d6c/1 -> Product_bc97e/2
  Constant_x_qdd_69022/1 -> Subtract_d1edb/2
  State_psi_kq_SG_D_1_494df/1 -> Product_f7217/1
  Constant_-1_b6810/1 -> Product_bc97e/1
  Constant_x_qd_82ebf/1 -> Subtract_d1edb/1
  State_psi_gq_SG_D_1_af930/1 -> Product_1b672/1
  Product_a14b6/1 -> Blockout_d_psi_q_SG_D_1_f8953/1
  Subtract_ba1bd/1 -> Add_3c619/1
  Product_1b672/1 -> Divide_2b1a9/1
  Add_97b80/1 -> Product_1b672/2
  Divide_4c773/1 -> Subtract_ba1bd/2
  Product_1c24e/1 -> Add_7d812/1
  Constant_x_qd_f92bb/1 -> Add_7d812/2
  Constant_-2.0_8fd1c/1 -> Product_cb3f5/1
  Product_f7217/1 -> Divide_4c773/1
  Product_bc97e/1 -> Add_16bac/1
  Subtract_d1edb/1 -> Product_f7217/2
  Constant_x_qd_2eb8b/1 -> Add_16bac/2
  Add_7d812/1 -> Divide_2b1a9/2
  Add_16bac/1 -> Divide_4c773/2
  Constant_f0_dc23e/1 -> Product_26d1a/2
  State_psi_q_SG_D_1_68044/1 -> Add_3c619/2
  Product_39025/1 -> Product_578ea/1
  Constant_R_a_cb351/1 -> Product_dbf66/1
  Product_578ea/1 -> Divide_fa36b/2
  Product_dbf66/1 -> Divide_0cb61/1
  Add_3c619/1 -> Product_dbf66/2
  State_theta_SG_D_1_16401/1 -> MathFunc_cos_1cdd6/1
  Input_v_d_SG_D_1_3462f/1 -> Product_fa442/1
  Constant_x_qdd_d1603/1 -> Divide_0cb61/2
  MathFunc_cos_1cdd6/1 -> Product_fa442/2
  State_theta_SG_D_1_4261b/1 -> MathFunc_sin_c5f98/1
  Divide_0cb61/1 -> Subtract_754fd/1
  Constant_2.0_360c5/1 -> Product_39025/1
  State_w_SG_D_1_856b5/1 -> Product_5e589/2
  Constant_pi_8069f/1 -> Product_39025/2
  Subtract_3f2ba/1 -> Add_3fe38/1
  Product_fa442/1 -> Subtract_754fd/2
  Divide_fa36b/1 -> Add_3fe38/2
  Input_v_q_SG_D_1_86d27/1 -> Product_c62d3/1
  MathFunc_sin_c5f98/1 -> Product_c62d3/2
  Product_c62d3/1 -> Subtract_3f2ba/2
  State_psi_d_SG_D_1_ad817/1 -> Product_5e589/1
  Constant_f0_165d7/1 -> Product_578ea/2
  Constant_pi_80d9b/1 -> Product_cb3f5/2
  Subtract_754fd/1 -> Subtract_3f2ba/1
  Product_5e589/1 -> Divide_fa36b/1
  Product_cb3f5/1 -> Product_26d1a/1
  Product_26d1a/1 -> Product_a14b6/1
  Add_3fe38/1 -> Product_a14b6/2

== system IEEE14_case/SG_D_1/d_theta_SG_D_1_block ==
  note: d_theta_SG_D_1 in case14gfl
      | $w_{\mathrm{SG},D,1}-2\,\pi \,f_{0}$
      | Automatically generated on 2025-10-09 21:30:13 .
  State_w_SG_D_1_d1dcd : Inport
  Add_3081f : Sum
  Constant_-2.0_8060a : Constant  Value=-2.0
  Constant_f0_111aa : Constant  Value=f0
  Constant_pi_f3045 : Constant  Value=pi
  Product_77390 : Product
  Product_fe15b : Product
  Blockout_d_theta_SG_D_1_10b81 : Outport
  wires:
  State_w_SG_D_1_d1dcd/1 -> Add_3081f/2
  Constant_-2.0_8060a/1 -> Product_fe15b/1
  Constant_f0_111aa/1 -> Product_77390/2
  Constant_pi_f3045/1 -> Product_fe15b/2
  Product_77390/1 -> Add_3081f/1
  Product_fe15b/1 -> Product_77390/1
  Add_3081f/1 -> Blockout_d_theta_SG_D_1_10b81/1

== system IEEE14_case/SG_D_1/d_w_SG_D_1_block ==
  note: d_w_SG_D_1 in case14gfl
      | $\frac{2\,\pi \,T_{m,\mathrm{SG},D,1}\,f_{0}-D\,\left(w_{\mathrm{SG},D,1}-2\,\pi \,f_{0}\right)+2\,\pi \,f_{0}\,\left(\frac{\psi _{d,\mathrm{SG},D,1}\,\left(\psi _{q,\mathrm{SG},D,1}+\frac{\psi _{\mathrm{gq},\mathrm{SG},D,1}\,\left(x_{l}-x_{\mathrm{qdd}}\right)}{x_{l}-x_{\mathrm{qd}}}+\frac{\psi _{\mathrm{kq},\mathrm{SG},D,1}\,\left(x_{\mathrm{qd}}-x_{\mathrm{qdd}}\right)}{x_{l}-x_{\mathrm{qd}}}\right)}{x_{\mathrm{qdd}}}+\frac{\psi _{q,\mathrm{SG},D,1}\,\left(\frac{\psi _{\mathrm{1d},\mathrm{SG},D,1}\,\left(x_{\mathrm{dd}}-x_{\mathrm{ddd}}\right)}{x_{\mathrm{dd}}-x_{l}}-\psi _{d,\mathrm{SG},D,1}+\frac{\psi _{\mathrm{fd},\mathrm{SG},D,1}\,\left(x_{\mathrm{ddd}}-x_{l}\right)}{x_{\mathrm{dd}}-x_{l}}\right)}{x_{\mathrm{ddd}}}\right)}{2\,H}$
      | Automatically generated on 2025-10-09 21:30:11 .
  State_w_SG_D_1_bf0fb : Inport
  State_T_m_SG_D_1_e0642 : Inport  Port=2
  State_psi_d_SG_D_1_3bbbe : Inport  Port=3
  State_psi_gq_SG_D_1_d212a : Inport  Port=4
  State_psi_kq_SG_D_1_9c615 : Inport  Port=5
  State_psi_q_SG_D_1_06dea : Inport  Port=6
  State_psi_q_SG_D_1_36eb9 : Inport  Port=7
  State_psi_1d_SG_D_1_bb43d : Inport  Port=8
  State_psi_d_SG_D_1_eab0d : Inport  Port=9
  State_psi_fd_SG_D_1_a5e83 : Inport  Port=10
  Add_0b580 : Sum
  Add_4d057 : Sum
  Add_50d54 : Sum
  Add_6bae3 : Sum
  Add_81276 : Sum
  Add_a641b : Sum
  Add_ba220 : Sum
  Add_ee1cf : Sum
  Constant_-1_1f6be : Constant  Value=-1
  Constant_-1_3c550 : Constant  Value=-1
  Constant_-1_46589 : Constant  Value=-1
  Constant_-1_64928 : Constant  Value=-1
  Constant_-1_97185 : Constant  Value=-1
  Constant_-1_b77df : Constant  Value=-1
  Constant_-2.0_6e9d5 : Constant  Value=-2.0
  Constant_2.0_5baea : Constant  Value=2.0
  Constant_2.0_82ce5 : Constant  Value=2.0
  Constant_2.0_d25e4 : Constant  Value=2.0
  Constant_D_1441e : Constant  Value=D
  Constant_H_ac4e4 : Constant  Value=H
  Constant_f0_26ca0 : Constant  Value=f0
  Constant_f0_34299 : Constant  Value=f0
  Constant_f0_41689 : Constant  Value=f0
  Constant_pi_84902 : Constant  Value=pi
  Constant_pi_a21ca : Constant  Value=pi
  Constant_pi_d7005 : Constant  Value=pi
  Constant_x_dd_92321 : Constant  Value=x_dd
  Constant_x_dd_b2cff : Constant  Value=x_dd
  Constant_x_dd_e9d04 : Constant  Value=x_dd
  Constant_x_ddd_022f1 : Constant  Value=x_ddd
  Constant_x_ddd_1dba0 : Constant  Value=x_ddd
  Constant_x_ddd_c68b2 : Constant  Value=x_ddd
  Constant_x_l_350b3 : Constant  Value=x_l
  Constant_x_l_42bf4 : Constant  Value=x_l
  Constant_x_l_89d86 : Constant  Value=x_l
  Constant_x_l_aee17 : Constant  Value=x_l
  Constant_x_l_b8821 : Constant  Value=x_l
  Constant_x_l_f6429 : Constant  Value=x_l
  Constant_x_qd_45fa0 : Constant  Value=x_qd
  Constant_x_qd_56588 : Constant  Value=x_qd
  Constant_x_qd_e35e2 : Constant  Value=x_qd
  Constant_x_qdd_353ea : Constant  Value=x_qdd
  Constant_x_qdd_e3224 : Constant  Value=x_qdd
  Constant_x_qdd_e6e28 : Constant  Value=x_qdd
  Divide_149e5 : Product  Inputs=*/
  Divide_40a9a : Product  Inputs=*/
  Divide_4168c : Product  Inputs=*/
  Divide_5bedd : Product  Inputs=*/
  Divide_d9125 : Product  Inputs=*/
  Divide_e4ce1 : Product  Inputs=*/
  Divide_f149a : Product  Inputs=*/
  Product_01f9b : Product
  Product_13840 : Product
  Product_27d64 : Product
  Product_2c9f5 : Product
  Product_354d4 : Product
  Product_3b237 : Product
  Product_3e25f : Product
  Product_43a3e : Product
  Product_67089 : Product
  Product_67f12 : Product
  Product_6b2db : Product
  Product_7d6ac : Product
  Product_93c17 : Product
  Product_94d69 : Product
  Product_b6f7f : Product
  Product_b75c0 : Product
  Product_b7bfa : Product
  Product_ce8e9 : Product
  Product_d1026 : Product
  Product_de552 : Product
  Product_f75d3 : Product
  Product_fa93d : Product
  Subtract_2cde9 : Sum  Inputs=+-
  Subtract_99796 : Sum  Inputs=+-
  Subtract_b4c93 : Sum  Inputs=+-
  Subtract_b54c6 : Sum  Inputs=+-
  Subtract_b9261 : Sum  Inputs=+-
  Subtract_bedff : Sum  Inputs=+-
  Subtract_e299b : Sum  Inputs=+-
  Subtract_fd590 : Sum  Inputs=+-
  Blockout_d_w_SG_D_1_3fcfa : Outport
  wires:
  Product_b6f7f/1 -> Add_ee1cf/1
  Constant_-1_1f6be/1 -> Product_b7bfa/1
  Constant_pi_d7005/1 -> Product_fa93d/2
  Constant_x_qdd_e6e28/1 -> Add_a641b/2
  Constant_x_l_b8821/1 -> Product_b7bfa/2
  Product_b7bfa/1 -> Add_a641b/1
  Constant_x_qd_56588/1 -> Subtract_99796/1
  Constant_-1_64928/1 -> Product_94d69/1
  Product_7d6ac/1 -> Product_b6f7f/1
  Constant_x_qdd_e3224/1 -> Subtract_99796/2
  State_psi_q_SG_D_1_36eb9/1 -> Product_3e25f/1
  Constant_x_l_89d86/1 -> Product_94d69/2
  Constant_-1_3c550/1 -> Product_67f12/1
  Constant_x_l_aee17/1 -> Product_67f12/2
  Constant_-1_b77df/1 -> Product_93c17/1
  Product_94d69/1 -> Add_4d057/1
  State_psi_1d_SG_D_1_bb43d/1 -> Product_93c17/2
  Constant_x_dd_92321/1 -> Subtract_b9261/1
  Subtract_99796/1 -> Product_f75d3/2
  Constant_x_ddd_c68b2/1 -> Subtract_b9261/2
  State_psi_gq_SG_D_1_d212a/1 -> Product_ce8e9/1
  Product_354d4/1 -> Product_13840/1
  Add_a641b/1 -> Product_ce8e9/2
  Constant_x_qd_45fa0/1 -> Add_4d057/2
  State_psi_kq_SG_D_1_9c615/1 -> Product_f75d3/1
  Constant_f0_26ca0/1 -> Product_b6f7f/2
  Product_67f12/1 -> Add_81276/1
  Constant_x_dd_e9d04/1 -> Subtract_b4c93/1
  Constant_x_qd_e35e2/1 -> Add_81276/2
  Product_93c17/1 -> Product_de552/1
  Subtract_b9261/1 -> Product_de552/2
  Constant_x_l_f6429/1 -> Subtract_b4c93/2
  Constant_x_ddd_1dba0/1 -> Subtract_bedff/1
  Constant_x_l_350b3/1 -> Subtract_bedff/2
  State_w_SG_D_1_bf0fb/1 -> Add_ee1cf/2
  Divide_5bedd/1 -> Add_6bae3/1
  Constant_-1_46589/1 -> Product_43a3e/1
  Product_ce8e9/1 -> Divide_f149a/1
  Add_ee1cf/1 -> Product_01f9b/2
  Divide_f149a/1 -> Subtract_e299b/1
  Add_4d057/1 -> Divide_f149a/2
  Constant_pi_84902/1 -> Product_7d6ac/2
  Product_f75d3/1 -> Divide_40a9a/1
  Add_81276/1 -> Divide_40a9a/2
  Product_de552/1 -> Divide_e4ce1/1
  Divide_e4ce1/1 -> Add_50d54/1
  Subtract_b4c93/1 -> Divide_e4ce1/2
  State_psi_fd_SG_D_1_a5e83/1 -> Product_b75c0/1
  Subtract_bedff/1 -> Product_b75c0/2
  Constant_x_dd_b2cff/1 -> Subtract_2cde9/1
  Constant_x_l_42bf4/1 -> Subtract_2cde9/2
  Divide_40a9a/1 -> Subtract_e299b/2
  Constant_2.0_5baea/1 -> Product_fa93d/1
  State_psi_d_SG_D_1_eab0d/1 -> Add_50d54/2
  Product_b75c0/1 -> Divide_4168c/1
  Subtract_2cde9/1 -> Divide_4168c/2
  Constant_-2.0_6e9d5/1 -> Product_7d6ac/1
  Constant_-1_97185/1 -> Product_354d4/1
  State_psi_d_SG_D_1_3bbbe/1 -> Product_354d4/2
  Subtract_e299b/1 -> Add_ba220/1
  Subtract_fd590/1 -> Product_3e25f/2
  State_psi_q_SG_D_1_06dea/1 -> Add_ba220/2
  Add_50d54/1 -> Subtract_fd590/1
  Divide_4168c/1 -> Subtract_fd590/2
  Add_ba220/1 -> Product_13840/2
  Constant_D_1441e/1 -> Product_43a3e/2
  Product_fa93d/1 -> Product_d1026/1
  State_T_m_SG_D_1_e0642/1 -> Product_d1026/2
  Constant_2.0_82ce5/1 -> Product_27d64/1
  Constant_pi_a21ca/1 -> Product_27d64/2
  Product_13840/1 -> Divide_5bedd/1
  Constant_x_qdd_353ea/1 -> Divide_5bedd/2
  Product_3e25f/1 -> Divide_d9125/1
  Constant_x_ddd_022f1/1 -> Divide_d9125/2
  Product_43a3e/1 -> Product_01f9b/1
  Product_d1026/1 -> Product_3b237/1
  Constant_f0_41689/1 -> Product_3b237/2
  Product_27d64/1 -> Product_2c9f5/1
  Constant_f0_34299/1 -> Product_2c9f5/2
  Divide_d9125/1 -> Add_6bae3/2
  Product_01f9b/1 -> Add_0b580/1
  Product_3b237/1 -> Add_0b580/2
  Product_2c9f5/1 -> Product_6b2db/1
  Add_6bae3/1 -> Product_6b2db/2
  Add_0b580/1 -> Subtract_b54c6/1
  Product_6b2db/1 -> Subtract_b54c6/2
  Constant_2.0_d25e4/1 -> Product_67089/1
  Constant_H_ac4e4/1 -> Product_67089/2
  Subtract_b54c6/1 -> Divide_149e5/1
  Product_67089/1 -> Divide_149e5/2
  Divide_149e5/1 -> Blockout_d_w_SG_D_1_3fcfa/1

== system IEEE14_case/SG_D_1/i_d_SG_D_1_block ==
  note: i_d_SG_D_1 in case14gfl
      | $\frac{\sin\left(\theta _{\mathrm{SG},D,1}\right)\,\left(\frac{\psi _{\mathrm{1d},\mathrm{SG},D,1}\,\left(x_{\mathrm{dd}}-x_{\mathrm{ddd}}\right)}{x_{\mathrm{dd}}-x_{l}}-\psi _{d,\mathrm{SG},D,1}+\frac{\psi _{\mathrm{fd},\mathrm{SG},D,1}\,\left(x_{\mathrm{ddd}}-x_{l}\right)}{x_{\mathrm{dd}}-x_{l}}\right)}{x_{\mathrm{ddd}}}-\frac{\cos\left(\theta _{\mathrm{SG},D,1}\right)\,\left(\psi _{q,\mathrm{SG},D,1}+\frac{\psi _{\mathrm{gq},\mathrm{SG},D,1}\,\left(x_{l}-x_{\mathrm{qdd}}\right)}{x_{l}-x_{\mathrm{qd}}}+\frac{\psi _{\mathrm{kq},\mathrm{SG},D,1}\,\left(x_{\mathrm{qd}}-x_{\mathrm{qdd}}\right)}{x_{l}-x_{\mathrm{qd}}}\right)}{x_{\mathrm{qdd}}}$
      | Automatically generated on 2025-10-09 21:30:31 .
  State_psi_gq_SG_D_1_8ae81 : Inport
  State_psi_kq_SG_D_1_0b4c3 : Inport  Port=2
  State_psi_q_SG_D_1_e8ece : Inport  Port=3
  State_theta_SG_D_1_02ca1 : Inport  Port=4
  State_psi_1d_SG_D_1_6fa9d : Inport  Port=5
  State_psi_d_SG_D_1_e218a : Inport  Port=6
  State_psi_fd_SG_D_1_51096 : Inport  Port=7
  State_theta_SG_D_1_8959d : Inport  Port=8
  Add_3be61 : Sum
  Add_4c251 : Sum
  Add_7b8bf : Sum
  Add_7dba2 : Sum
  Add_f3ef8 : Sum
  Constant_-1_2c4b9 : Constant  Value=-1
  Constant_-1_6a3e6 : Constant  Value=-1
  Constant_-1_a27e5 : Constant  Value=-1
  Constant_-1_b6280 : Constant  Value=-1
  Constant_-1_d576b : Constant  Value=-1
  Constant_x_dd_1c293 : Constant  Value=x_dd
  Constant_x_dd_e7313 : Constant  Value=x_dd
  Constant_x_dd_e8314 : Constant  Value=x_dd
  Constant_x_ddd_23677 : Constant  Value=x_ddd
  Constant_x_ddd_6de1c : Constant  Value=x_ddd
  Constant_x_ddd_a905f : Constant  Value=x_ddd
  Constant_x_l_1bce6 : Constant  Value=x_l
  Constant_x_l_6ab04 : Constant  Value=x_l
  Constant_x_l_a73a2 : Constant  Value=x_l
  Constant_x_l_abe1a : Constant  Value=x_l
  Constant_x_l_be453 : Constant  Value=x_l
  Constant_x_l_da08f : Constant  Value=x_l
  Constant_x_qd_2e4f8 : Constant  Value=x_qd
  Constant_x_qd_63b02 : Constant  Value=x_qd
  Constant_x_qd_93e3b : Constant  Value=x_qd
  Constant_x_qdd_3694c : Constant  Value=x_qdd
  Constant_x_qdd_90caa : Constant  Value=x_qdd
  Constant_x_qdd_bc76a : Constant  Value=x_qdd
  Divide_19587 : Product  Inputs=*/
  Divide_38676 : Product  Inputs=*/
  Divide_a9eb6 : Product  Inputs=*/
  Divide_c2f05 : Product  Inputs=*/
  Divide_ed0f1 : Product  Inputs=*/
  Divide_fbbe9 : Product  Inputs=*/
  MathFunc_cos_ea059 : Trigonometry  Operator=cos
  MathFunc_sin_5b8f4 : Trigonometry
  Product_26c62 : Product
  Product_454aa : Product
  Product_51457 : Product
  Product_585ae : Product
  Product_5f1a1 : Product
  Product_85bd2 : Product
  Product_af2b7 : Product
  Product_bd21e : Product
  Product_c1c0f : Product
  Product_d03bf : Product
  Product_d4172 : Product
  Subtract_45d88 : Sum  Inputs=+-
  Subtract_71db4 : Sum  Inputs=+-
  Subtract_779af : Sum  Inputs=+-
  Subtract_784db : Sum  Inputs=+-
  Subtract_85519 : Sum  Inputs=+-
  Subtract_8edb7 : Sum  Inputs=+-
  Subtract_9a956 : Sum  Inputs=+-
  Subtract_c9a44 : Sum  Inputs=+-
  Blockout_i_d_SG_D_1_f5e95 : Outport
  wires:
  Constant_-1_d576b/1 -> Product_5f1a1/1
  Constant_x_l_6ab04/1 -> Product_5f1a1/2
  Constant_x_ddd_a905f/1 -> Subtract_779af/2
  Product_5f1a1/1 -> Add_f3ef8/1
  Constant_x_qdd_3694c/1 -> Subtract_45d88/2
  Constant_x_l_abe1a/1 -> Product_c1c0f/2
  Constant_x_qd_2e4f8/1 -> Add_7b8bf/2
  Constant_x_qdd_90caa/1 -> Add_f3ef8/2
  Constant_x_qd_63b02/1 -> Subtract_45d88/1
  MathFunc_cos_ea059/1 -> Product_d4172/2
  Constant_-1_6a3e6/1 -> Product_c1c0f/1
  Constant_-1_b6280/1 -> Product_454aa/1
  Subtract_71db4/1 -> Blockout_i_d_SG_D_1_f5e95/1
  Constant_x_l_a73a2/1 -> Product_454aa/2
  Divide_ed0f1/1 -> Subtract_c9a44/1
  State_psi_gq_SG_D_1_8ae81/1 -> Product_85bd2/1
  Subtract_85519/1 -> Product_585ae/2
  Add_f3ef8/1 -> Product_85bd2/2
  Divide_fbbe9/1 -> Add_3be61/1
  Product_c1c0f/1 -> Add_4c251/1
  Constant_x_qd_93e3b/1 -> Add_4c251/2
  State_psi_kq_SG_D_1_0b4c3/1 -> Product_51457/1
  Add_3be61/1 -> Subtract_9a956/1
  Add_4c251/1 -> Divide_ed0f1/2
  Subtract_45d88/1 -> Product_51457/2
  Product_454aa/1 -> Add_7b8bf/1
  Constant_-1_2c4b9/1 -> Product_26c62/1
  State_psi_1d_SG_D_1_6fa9d/1 -> Product_26c62/2
  Constant_x_dd_e7313/1 -> Subtract_779af/1
  Product_85bd2/1 -> Divide_ed0f1/1
  Product_d03bf/1 -> Divide_19587/1
  Subtract_779af/1 -> Product_bd21e/2
  Product_51457/1 -> Divide_38676/1
  Product_26c62/1 -> Product_bd21e/1
  Add_7b8bf/1 -> Divide_38676/2
  Constant_x_dd_e8314/1 -> Subtract_784db/1
  Subtract_c9a44/1 -> Add_7dba2/1
  Constant_x_l_1bce6/1 -> Subtract_784db/2
  Constant_x_ddd_6de1c/1 -> Subtract_85519/1
  Constant_x_l_da08f/1 -> Subtract_85519/2
  Divide_19587/1 -> Subtract_71db4/2
  Divide_38676/1 -> Subtract_c9a44/2
  State_theta_SG_D_1_02ca1/1 -> MathFunc_cos_ea059/1
  Product_bd21e/1 -> Divide_fbbe9/1
  Subtract_784db/1 -> Divide_fbbe9/2
  State_theta_SG_D_1_8959d/1 -> MathFunc_sin_5b8f4/1
  State_psi_fd_SG_D_1_51096/1 -> Product_585ae/1
  Constant_x_dd_1c293/1 -> Subtract_8edb7/1
  Constant_x_l_be453/1 -> Subtract_8edb7/2
  State_psi_q_SG_D_1_e8ece/1 -> Add_7dba2/2
  State_psi_d_SG_D_1_e218a/1 -> Add_3be61/2
  Constant_x_ddd_23677/1 -> Divide_19587/2
  MathFunc_sin_5b8f4/1 -> Product_d03bf/2
  Product_585ae/1 -> Divide_c2f05/1
  Constant_-1_a27e5/1 -> Product_af2b7/1
  Subtract_8edb7/1 -> Divide_c2f05/2
  Add_7dba2/1 -> Product_af2b7/2
  Divide_c2f05/1 -> Subtract_9a956/2
  Product_af2b7/1 -> Product_d4172/1
  Subtract_9a956/1 -> Product_d03bf/1
  Constant_x_qdd_bc76a/1 -> Divide_a9eb6/2
  Product_d4172/1 -> Divide_a9eb6/1
  Divide_a9eb6/1 -> Subtract_71db4/1
